simulink model "IEEE9_16b_Rockefeller_uderen"  (R2020a)
settings: Solver=ode8  StartTime=0.0  StopTime=5  MaxStep=1e-4  RelTol=1e-3
undefined symbols (not defined in the file or in its folder): k
libraries: powerlib x33, powerlib_meascontrol x27, simulink_extras x24, dspsigops x6, sps_avr x3
(part 1 of 2)
settings Model: Creator=Pankaj  LastModifiedBy=ahmed
settings DataIOCC: ReturnWorkspaceOutputs=off
settings DebuggingCC: UnconnectedInputMsg=none  UnconnectedOutputMsg=none  UnconnectedLineMsg=none  ArithmeticOperatorsInVariantConditions=warning
settings SFSimCC: SimUseLocalCustomCode=off  CustomCodeUndefinedFunction=UseInterfaceOnly
settings RTWCC: RTWUseLocalCustomCode=off
settings CodeAppCC: StateflowObjectComments=on
settings SimscapeCC: SimscapeNormalizeSystem=off

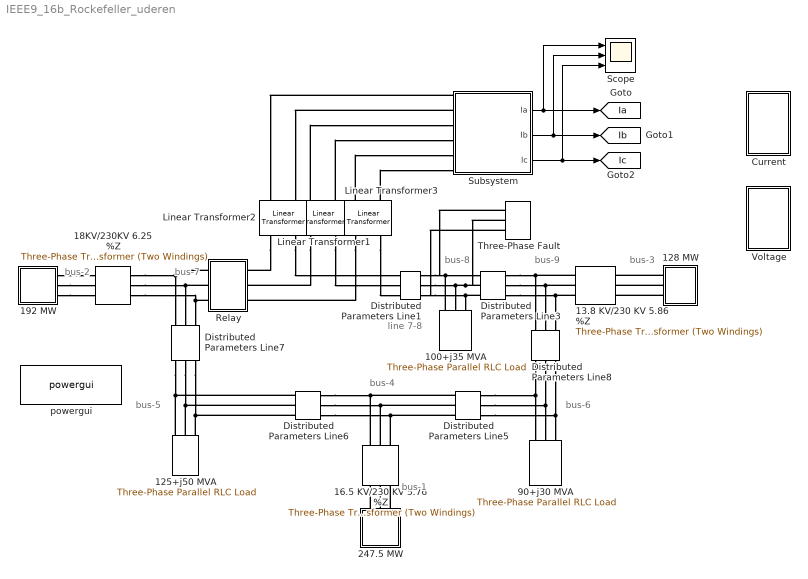
== system IEEE9_16b_Rockefeller_uderen ==
  note: bus-2
  note: bus-7
  note: bus-8
  note: bus-9
  note: bus-1
  note: bus-3
  note: bus-4
  note: bus-6
  note: bus-5
  note: line 7-8
  100+j35 MVA : powerlib/Elements/Three-Phase Parallel RLC Load  LConnTagsString=A|B|C  Configuration=Y (grounded)  NominalVoltage=(230000)*0.993698  Vabc=[1e3 1e3 1e3]  Vabcp=[1e3 1e3 1e3]  NominalFrequency=60  UnbalancedPower=off  ActivePower=100e6  InductivePower=35e6  CapacitivePower=0  Pabc=[10e3 9e3 11e3]  QLabc=[100 90 110]  QCabc=[100 90 110]  Pabcp=[10e3 9e3 11e3]  QLabcp=[100 90 110]  QCabcp=[100 90 110]  Measurements=None  LoadType=constant PQ
  125+j50 MVA : powerlib/Elements/Three-Phase Parallel RLC Load  LConnTagsString=A|B|C  Configuration=Y (grounded)  NominalVoltage=(223027)*1  Vabc=[1e3 1e3 1e3]  Vabcp=[1e3 1e3 1e3]  NominalFrequency=60  UnbalancedPower=off  ActivePower=125e6  InductivePower=50e6  CapacitivePower=0  Pabc=[10e3 9e3 11e3]  QLabc=[100 90 110]  QCabc=[100 90 110]  Pabcp=[10e3 9e3 11e3]  QLabcp=[100 90 110]  QCabcp=[100 90 110]  Measurements=None  LoadType=constant PQ
  128 MW : Subsystem
  13.8 KV/230 KV 5.86 %Z : powerlib/Elements/Three-Phase Transformer (Two Windings)  Winding1Connection=Yg  Winding2Connection=Yg  CoreType=Three single-phase transformers  SetSaturation=off  Hysteresis=off  DataFile='hysteresis'  SetInitialFlux=off  Measurements=None  UNITS=pu  NominalPower=[ 100e6 , 60 ]  Winding1=[13.8e3 , 1e-6 , 0 ]  Winding2=[ 230e3 , 1e-6, 0.0586 ]  Rm=500  Lm=500  L0=0.5  Saturation=[ 0,0 ; 0.0024,1.2 ; 1.0,1.52 ]  InitialFluxes=[ 0.8 , -0.8 , 0.7 ]  BreakLoop=off  DiscreteSolver=Trapezoidal iterative  DataType=off  TransfoNumber=1
  "16.5 KV/230 KV 5.76 %Z     " : powerlib/Elements/Three-Phase Transformer (Two Windings)  Winding1Connection=Yg  Winding2Connection=Yg  CoreType=Three single-phase transformers  SetSaturation=off  Hysteresis=off  DataFile='hysteresis'  SetInitialFlux=off  Measurements=None  UNITS=pu  NominalPower=[ 100e6 , 60 ]  Winding1=[16.5e3 , 1e-6, 0 ]  Winding2=[ 230e3 ,1e-6, 0.0576 ]  Rm=500  Lm=500  L0=0.5  Saturation=[ 0,0 ; 0.0024,1.2 ; 1.0,1.52 ]  InitialFluxes=[ 0.8 , -0.8 , 0.7 ]  BreakLoop=off  DiscreteSolver=Trapezoidal iterative  DataType=off  TransfoNumber=1
  18KV/230KV 6.25 %Z : powerlib/Elements/Three-Phase Transformer (Two Windings)  Winding1Connection=Yg  Winding2Connection=Yg  CoreType=Three single-phase transformers  SetSaturation=off  Hysteresis=off  DataFile='hysteresis'  SetInitialFlux=off  Measurements=None  UNITS=pu  NominalPower=[ 100e6 , 60 ]  Winding1=[ 18e3 , 1e-6 , 0]  Winding2=[ 230e3 , 1e-6, 0.0625 ]  Rm=500  Lm=500  L0=0.5  Saturation=[ 0,0 ; 0.0024,1.2 ; 1.0,1.52 ]  InitialFluxes=[ 0.8 , -0.8 , 0.7 ]  BreakLoop=off  DiscreteSolver=Trapezoidal iterative  DataType=off  TransfoNumber=1
  192 MW : Subsystem
  247.5 MW : Subsystem
  90+j30 MVA : powerlib/Elements/Three-Phase Parallel RLC Load  LConnTagsString=A|B|C  Configuration=Y (grounded)  NominalVoltage=(226177)*0.999999  Vabc=[1e3 1e3 1e3]  Vabcp=[1e3 1e3 1e3]  NominalFrequency=60  UnbalancedPower=off  ActivePower=90e6  InductivePower=30e6  CapacitivePower=0  Pabc=[10e3 9e3 11e3]  QLabc=[100 90 110]  QCabc=[100 90 110]  Pabcp=[10e3 9e3 11e3]  QLabcp=[100 90 110]  QCabcp=[100 90 110]  Measurements=None  LoadType=constant PQ
  "Current " : Subsystem
  Distributed Parameters Line1 : powerlib/Elements/Distributed Parameters Line  Phases=3  Frequency=60  Resistance=[0.044965 0.11241]  Inductance="[1.01e-3  2.02e-3]"  Capacitance=[12.74e-9 7.751e-9]  Length=100  x1=[-0.000416666666666667 4.03999386636865e-10 0 0;-0.000388888888888889 4.03567307365848e-10 0 0;-0.000361111111111111 4.03090972391788e-10 75770.798481712 -217642.762175141;-0.000333333333333333 4.02570433950183e-10 78045.7469011949 -216837.371769227;-0.000305555555555556 4.02005749123939e-10 80312.1367250346 -216008.202701964;-0.000277777777777778 4.0139697983711e-10 82569.7194180468 -215155.345901084;-0.00025 4.0074419284811e-10 84818.2474108487 -214278.894891945;-0.000222222222222222 4.00047459742387e-10 87057.4741270072 -213378.945787278;-0.000194444444444444 3.99306856924578e-10 89287.1540100791 -212455.597276643;-0.000166666666666667 3.98522465610128e-10 91507.042550539 -211508.950615609;-0.000138888888888889 3.97694371816383e-10 93716.8963125926 -210539.109614652;-0.000111111111111111 3.96822666353162e-10 95916.4729608721 -209546.180627764;-8.33333333333333e-05 3.95907444812789e-10 98105.5312870111 -208530.272540801;-5.55555555555556e-05 3.94948807559621e-10 100283.831236096 -207491.49675953;-2.77777777777778e-05 3.93946859719036e-10 102451.133932989 -206429.967197424]  x2=[-0.000416666666666667 2.24406788779024e-10 0 0;-0.000388888888888889 2.22220992142664e-10 0 0;-0.000361111111111111 2.20010826470313e-10 65495.6415441537 -218920.534617487;-0.000333333333333333 2.17776534131542e-10 67784.5337476624 -218222.674162098;-0.000305555555555556 2.15518360141686e-10 70065.9926131833 -217500.88313134;-0.000277777777777778 2.13236552134969e-10 72339.7679530423 -216755.240677735;-0.00025 2.10931360337352e-10 74605.6104221501 -215985.82856938;-0.000222222222222222 2.08603037539095e-10 76863.2715453463 -215192.731180984;-0.000194444444444444 2.06251839067028e-10 79112.5037446472 -214376.035484611;-0.000166666666666667 2.03878022756561e-10 81353.0603663957 -213535.83104015;-0.000138888888888889 2.01481848923403e-10 83584.6957083093 -212672.209985485;-0.000111111111111111 1.99063580335015e-10 85807.1650464246 -211785.267026397;-8.33333333333333e-05 1.96623482181802e-10 88020.2246619337 -210875.099426176;-5.55555555555556e-05 1.94161822048021e-10 90223.6318679107 -209941.806994957;-2.77777777777778e-05 1.91678869882449e-10 92417.1450359256 -208985.492078772]  x3=[-0.000416666666666667 2.4657287812106e-12 0 0;-0.000388888888888889 2.44181675130627e-12 0 0;-0.000361111111111111 2.41763694867838e-12 149.88034762837 -520.868275171293;-0.000333333333333333 2.39319202491478e-12 155.326551453273 -519.270203705918;-0.000305555555555556 2.36848466067682e-12 160.755721971439 -517.615188411064;-0.000277777777777778 2.34351756540542e-12 166.167263813138 -515.903410777807;-0.00025 2.31829347702393e-12 171.560583541825 -514.135058521855;-0.000222222222222222 2.2928151616379e-12 176.935089719215 -512.310325562961;-0.000194444444444444 2.26708541323171e-12 182.29019297014 -510.429412003656;-0.000166666666666667 2.24110705336223e-12 187.625306047182 -508.492524107308;-0.000138888888888889 2.21488293084937e-12 192.93984389507 -506.499874275502;-0.000111111111111111 2.18841592146368e-12 198.233223714842 -504.451681024747;-8.33333333333333e-05 2.161708927611e-12 203.504865027747 -502.348168962514;-5.55555555555556e-05 2.13476487801416e-12 208.754189738911 -500.189568762605;-2.77777777777778e-05 2.10758672739183e-12 213.980622200724 -497.976117139856]  x4=[-0.000416666666666667 -9.98914374453805e-13 0 0;-0.000388888888888889 -9.81740072469835e-13 0 0;-0.000361111111111111 -9.64458111623713e-13 241.700354629401 -1044.85957766127;-0.000333333333333333 -9.47070387077197e-13 252.628607776882 -1042.27124557573;-0.000305555555555556 -9.29578805590225e-13 263.529157350655 -1039.56861670278;-0.000277777777777778 -9.11985285311819e-13 274.40080798262 -1036.75198741614;-0.00025 -8.94291755569738e-13 285.242367473774 -1033.82166659095;-0.000222222222222222 -8.76500156658907e-13 296.052646924945 -1030.7779755699;-0.000194444444444444 -8.58612439628639e-13 306.830460867171 -1027.62124812802;-0.000166666666666667 -8.40630566068683e-13 317.574627391698 -1024.35183043604;-0.000138888888888889 -8.22556507894113e-13 328.28396827959 -1020.97008102246;-0.000111111111111111 -8.04392247129082e-13 338.957309130937 -1017.47637073421;-8.33333333333333e-05 -7.86139775689477e-13 349.593479493636 -1013.87108269599;-5.55555555555556e-05 -7.67801095164478e-13 360.191312991747 -1010.15461226827;-2.77777777777778e-05 -7.49378216597062e-13 370.749647453402 -1006.3273670039]  x5=0.000395689524753941  V1=[5.416e-10 2.305e+05 2.305e+05;377 377 377;2.885 0.3359 -1.235]  V2=[2.789e-10 2.285e+05 2.285e+05;377 377 377;2.728 0.2916 -1.279]  I1=[3.179e-12 542 542;377 377 377;-1.76 0.2811 -1.29]  I2=[4.124e-12 1072 1072;377 377 377;1.614 0.2282 -1.343]  nHarmo=1  Measurements=None
  Distributed Parameters Line3 : powerlib/Elements/Distributed Parameters Line  Phases=3  Frequency=60  Resistance=[ 0.062951 0.15737]  Inductance="[ 1.414e-3  3.53e-3]"  Capacitance=[12.74e-9 7.751e-9]  Length=100  x1=[-0.000527777777777778 2.32901531654904e-10 0 0;-0.0005 2.30815581018941e-10 0 0;-0.000472222222222222 2.28704318853463e-10 0 0;-0.000444444444444444 2.2656797668216e-10 58586.8788444457 -220869.780420169;-0.000416666666666667 2.24406788779024e-10 60896.5619220916 -220244.16032176;-0.000388888888888889 2.22220992142664e-10 63199.5670054809 -219594.387969246;-0.000361111111111111 2.20010826470313e-10 65495.6415441537 -218920.534617487;-0.000333333333333333 2.17776534131542e-10 67784.5337476624 -218222.674162098;-0.000305555555555556 2.15518360141686e-10 70065.9926131833 -217500.88313134;-0.000277777777777778 2.13236552134969e-10 72339.7679530423 -216755.240677735;-0.00025 2.10931360337352e-10 74605.6104221501 -215985.82856938;-0.000222222222222222 2.08603037539095e-10 76863.2715453463 -215192.731180984;-0.000194444444444444 2.06251839067028e-10 79112.5037446472 -214376.035484611;-0.000166666666666667 2.03878022756561e-10 81353.0603663957 -213535.83104015;-0.000138888888888889 2.01481848923403e-10 83584.6957083093 -212672.209985485;-0.000111111111111111 1.99063580335015e-10 85807.1650464246 -211785.267026397;-8.33333333333333e-05 1.96623482181802e-10 88020.2246619337 -210875.099426176;-5.55555555555556e-05 1.94161822048021e-10 90223.6318679107 -209941.806994957;-2.77777777777778e-05 1.91678869882449e-10 92417.1450359256 -208985.492078772]  x2=[-0.000527777777777778 3.2700270716933e-10 0 0;-0.0005 3.25421192626044e-10 0 0;-0.000472222222222222 3.23803991981823e-10 0 0;-0.000444444444444444 3.22151282580942e-10 67656.3360068027 -221170.891319713;-0.000416666666666667 3.20463245661611e-10 69968.6747078772 -220450.281883491;-0.000388888888888889 3.187400663361e-10 72273.3405552948 -219705.497589611;-0.000361111111111111 3.16981933570442e-10 74570.0808164739 -218936.620112065;-0.000333333333333333 3.15189040163706e-10 76858.6436279632 -218143.733766932;-0.000305555555555556 3.13361582726859e-10 79138.7780230604 -217326.925503135;-0.000277777777777778 3.11499761661201e-10 81410.2339593343 -216486.284892905;-0.00025 3.09603781136394e-10 83672.7623460448 -215621.904121957;-0.000222222222222222 3.07673849068068e-10 85926.1150714576 -214733.877979385;-0.000194444444444444 3.05710177095022e-10 88170.0450300536 -213822.303847261;-0.000166666666666667 3.03712980556018e-10 90404.3061496259 -212887.281689962;-0.000138888888888889 3.01682478466161e-10 92628.6534182649 -211928.914043204;-0.000111111111111111 2.99618893492888e-10 94842.8429112266 -210947.306002799;-8.33333333333333e-05 2.97522451931545e-10 97046.6318176814 -209942.565213131;-5.55555555555556e-05 2.95393383680575e-10 99239.7784673413 -208914.80185535;-2.77777777777778e-05 2.93231922216303e-10 101422.042356962 -207864.12863529]  x3=[-0.000527777777777778 5.83625832453338e-13 0 0;-0.0005 5.86026533236036e-13 0 0;-0.000472222222222222 5.88362969605446e-13 0 0;-0.000444444444444444 5.90634885344991e-13 134.791474574619 -835.193347915332;-0.000416666666666667 5.92842031313507e-13 143.530042644098 -833.736052248476;-0.000388888888888889 5.94984165472567e-13 152.252871026964 -832.18732802814;-0.000361111111111111 5.97061052913021e-13 160.959003166788 -830.547345089386;-0.000333333333333333 5.99072465880757e-13 169.647484338072 -828.816283274826;-0.000305555555555556 6.01018183801675e-13 178.317361750944 -826.994332414893;-0.000277777777777778 6.02897993305881e-13 186.967684655647 -825.081692307033;-0.00025 6.04711688251078e-13 195.597504446793 -823.078572693785;-0.000222222222222222 6.06459069745176e-13 204.205874767392 -820.985193239789;-0.000194444444444444 6.08139946168105e-13 212.791851612633 -818.801783507692;-0.000166666666666667 6.09754133192822e-13 221.354493433398 -816.528582932976;-0.000138888888888889 6.11301453805529e-13 229.892861239519 -814.165840797701;-0.000111111111111111 6.12781738325086e-13 238.406018702749 -811.713816203167;-8.33333333333333e-05 6.14194824421613e-13 246.893032259436 -809.172778041503;-5.55555555555556e-05 6.15540557134295e-13 255.352971212904 -806.543004966179;-2.77777777777778e-05 6.16818788888377e-13 263.784907835512 -803.824785361446]  x4=[-0.000527777777777778 7.12462384982262e-13 0 0;-0.0005 7.0072342704295e-13 0 0;-0.000472222222222222 6.88907626883427e-13 0 0;-0.000444444444444444 6.77016280239333e-13 133.427230259186 -503.056878765156;-0.000416666666666667 6.6505069113083e-13 138.687791245764 -501.632070106391;-0.000388888888888889 6.53012171719605e-13 143.933143553162 -500.15225183826;-0.000361111111111111 6.40902042164973e-13 149.16271196939 -498.61758623951;-0.000333333333333333 6.28721630479108e-13 154.375923013341 -497.028241603521;-0.000305555555555556 6.16472272381411e-13 159.572204997674 -495.38439221984;-0.000277777777777778 6.04155311152038e-13 164.750988091513 -493.686218355078;-0.00025 5.91772097484584e-13 169.911704382934 -491.933906233135;-0.000222222222222222 5.79323989337977e-13 175.053787941238 -490.127648014782;-0.000194444444444444 5.6681235178755e-13 180.176674879018 -488.267641776588;-0.000166666666666667 5.54238556875355e-13 185.279803413991 -486.354091489197;-0.000138888888888889 5.41603983459698e-13 190.362613930605 -484.387206994961;-0.000111111111111111 5.28910017063932e-13 195.424549041411 -482.367203984931;-8.33333333333333e-05 5.16158049724521e-13 200.465053648179 -480.2943039752;-5.55555555555556e-05 5.03349479838386e-13 205.483575002779 -478.168734282613;-2.77777777777778e-05 4.90485712009553e-13 210.479562767791 -475.99072799984]  x5=0.000523077718890797  V1=[2.541e-10 2.285e+05 2.285e+05;377 377 377;2.713 0.2668 -1.304]  V2=[4.31e-10 2.313e+05 2.313e+05;377 377 377;2.564 0.3044 -1.266]  I1=[1.418e-12 846 846;377 377 377;1.513 0.1676 -1.403]  I2=[2.062e-12 520.4 520.5;377 377 377;-2.991 0.2668 -1.304]  nHarmo=1  Measurements=None
  Distributed Parameters Line5 : powerlib/Elements/Distributed Parameters Line  Phases=3  Frequency=60  Resistance=[ 0.08993 0.224825]  Inductance="[ 1.29e-3  3.22e-3]"  Capacitance=[12.74e-9 7.751e-9]  Length=100  x1=[-0.0005 1.0080475529374e-10 59236.9573250748 -221110.335723773;-0.000472222222222222 9.85184782910845e-11 61549.1238482215 -220477.894229562;-0.000444444444444444 9.62213976270818e-11 63854.5408163426 -219821.274849687;-0.000416666666666667 9.39137652025128e-11 66152.955414488 -219140.549589866;-0.000388888888888889 9.15958340752774e-11 68444.1155955961 -218435.793099292;-0.000361111111111111 8.92678584326443e-11 70727.7701081341 -217707.082662457;-0.000333333333333333 8.69300935633769e-11 73003.6685236502 -216954.498190672;-0.000305555555555556 8.4582795829737e-11 75271.5612642361 -216178.122213305;-0.000277777777777778 8.2226222639373e-11 77531.199629896 -215378.039868732;-0.00025 7.98606324170912e-11 79782.3358258193 -214554.338894998;-0.000222222222222222 7.74862845765174e-11 82024.722989554 -213707.109620196;-0.000194444444444444 7.51034394916487e-11 84258.1152180784 -212836.444952564;-0.000166666666666667 7.2712358468301e-11 86482.2675947664 -211942.440370294;-0.000138888888888889 7.03133037154533e-11 88696.9362162461 -211025.193911063;-0.000111111111111111 6.79065383164944e-11 90901.878219146 -210084.806161282;-8.33333333333333e-05 6.54923262003719e-11 93096.8518067282 -209121.380245065;-5.55555555555556e-05 6.30709321126501e-11 95281.6162754036 -208135.02181292;-2.77777777777778e-05 6.06426215864773e-11 97455.9320411281 -207125.839030165]  x2=[-0.0005 3.88349738495921e-11 47819.8765851152 -221024.854138414;-0.000472222222222222 3.75142302196108e-11 50131.7738988869 -220511.975319648;-0.000444444444444444 3.6189372731539e-11 52438.1736987168 -219974.914877845;-0.000416666666666667 3.486054667093e-11 54738.8230618762 -219413.731707732;-0.000388888888888889 3.35278977585359e-11 57033.4696962363 -218828.48734937;-0.000361111111111111 3.21915721343275e-11 59321.8619679355 -218219.245981397;-0.000333333333333333 3.08517163414685e-11 61603.7489289732 -217586.074413995;-0.000305555555555556 2.95084773102454e-11 63878.8803447298 -216929.042081562;-0.000277777777777778 2.8162002341955e-11 66147.0067214069 -216248.221035096;-0.00025 2.68124390927508e-11 68407.8793333881 -215543.685934297;-0.000222222222222222 2.54599355574514e-11 70661.2502505137 -214815.514039379;-0.000194444444444444 2.41046400533108e-11 72906.8723652693 -214063.785202596;-0.000166666666666667 2.27467012037536e-11 75144.4994198843 -213288.581859486;-0.000138888888888889 2.13862679220775e-11 77373.8860333364 -212489.989019831;-0.000111111111111111 2.00234893951224e-11 79594.7877282605 -211668.094258336;-8.33333333333333e-05 1.86585150669109e-11 81806.9609577585 -210822.987705023;-5.55555555555556e-05 1.72914946222599e-11 84010.1631321068 -209954.762035348;-2.77777777777778e-05 1.59225779703662e-11 86204.1526453591 -209063.512460042]  x3=[-0.0005 -7.50982334861951e-13 90.1297776583444 -469.287337824947;-0.000472222222222222 -7.61225065980247e-13 95.0391104187908 -468.317788550188;-0.000444444444444444 -7.71384320191832e-13 99.9380210697864 -467.296882952453;-0.000416666666666667 -7.81458983419997e-13 104.825972390573 -466.224732985545;-0.000388888888888889 -7.91447950864387e-13 109.702428362205 -465.101456222789;-0.000361111111111111 -8.01350127122157e-13 114.566854226333 -463.927175844142;-0.000333333333333333 -8.11164426308094e-13 119.418716543844 -462.70202062268;-0.000305555555555556 -8.20889772173693e-13 124.25748325336 -461.426124910478;-0.000277777777777778 -8.30525098225186e-13 129.082623729582 -460.09962862388;-0.00025 -8.40069347840492e-13 133.893608841484 -458.722677228152;-0.000222222222222222 -8.49521474385086e-13 138.689911010332 -457.295421721531;-0.000194444444444444 -8.58880441326777e-13 143.471004267544 -455.818018618667;-0.000166666666666667 -8.68145222349374e-13 148.236364312368 -454.29062993346;-0.000138888888888889 -8.77314801465232e-13 152.985468569372 -452.71342316129;-0.000111111111111111 -8.86388173126671e-13 157.717796245759 -451.086571260654;-8.33333333333333e-05 -8.95364342336239e-13 162.432828388469 -449.410252634196;-5.55555555555556e-05 -9.04242324755831e-13 167.130047941094 -447.684651109143;-2.77777777777778e-05 -9.13021146814629e-13 171.808939800579 -445.909955917148]  x4=[-0.0005 1.03748190399177e-12 134.355884883261 -916.40247338539;-0.000472222222222222 1.03354240972687e-12 143.944855500255 -914.945276234842;-0.000444444444444444 1.02948957588978e-12 153.518040941732 -913.387745024259;-0.000416666666666667 1.02532384691939e-12 163.074391400029 -911.73005055449;-0.000388888888888889 1.02104567963485e-12 172.612858913627 -909.972374610413;-0.000361111111111111 1.01665554318539e-12 182.132397482076 -908.114909941004;-0.000333333333333333 1.01215391899896e-12 191.631963180695 -906.157860238195;-0.000305555555555556 1.00754130072936e-12 201.110514275055 -904.10144011454;-0.000277777777777778 1.00281819420219e-12 210.567011335215 -901.945875079679;-0.00025 9.97985117359288e-13 220.000417349708 -899.69140151561;-0.000222222222222222 9.93042600201997e-13 229.40969783926 -897.338266650764;-0.000194444444444444 9.8799118473302e-13 238.793820970231 -894.886728532896;-0.000166666666666667 9.8283142489699e-13 248.15175766777 -892.337056000788;-0.000138888888888889 9.77563886519715e-13 257.482481728666 -889.689528654765;-0.000111111111111111 9.7218914724614e-13 266.784969933876 -886.944436826035;-8.33333333333333e-05 9.66707796476994e-13 276.058202160739 -884.102081544852;-5.55555555555556e-05 9.61120435304157e-13 285.301161494842 -881.162774507502;-2.77777777777778e-05 9.55427676444746e-13 294.512834341536 -878.126838042126]  x5=0.000499582025297148  V1=[3.29e-10 2.289e+05 2.289e+05;377 377 377;2.341 0.2974 -1.273]  V2=[3.35e-10 2.261e+05 2.261e+05;377 377 377;2.353 0.2487 -1.322]  I1=[9.5e-13 477.9 477.9;377 377 377;2.529 0.2254 -1.345]  I2=[6.245e-14 926.2 926.2;377 377 377;-2.223 0.1812 -1.39]  nHarmo=1  Measurements=None
  Distributed Parameters Line6 : powerlib/Elements/Distributed Parameters Line  Phases=3  Frequency=60  Resistance=[ 0.0529 0.13225]  Inductance="[ 1.192e-3  2.38e-3]"  Capacitance=[12.74e-9 7.751e-9]  Length=100  x1=[-0.000444444444444444 2.06940842119763e-10 0 0;-0.000416666666666667 2.06909650746566e-10 51040.896855504 -217071.807600682;-0.000388888888888889 2.06855769398504e-10 53311.2223029157 -216525.415158399;-0.000361111111111111 2.06779203984275e-10 55575.7015740392 -215955.278264325;-0.000333333333333333 2.06679962900139e-10 57834.0863432037 -215361.459440394;-0.000305555555555556 2.06558057029e-10 60086.1289530699 -214744.023805532;-0.000277777777777778 2.0641349973921e-10 62331.5824417872 -214103.039068515;-0.00025 2.06246306883104e-10 64570.2005700766 -213438.575520542;-0.000222222222222222 2.06056496795265e-10 66801.7378482336 -212750.706027529;-0.000194444444444444 2.05844090290506e-10 69025.9495630483 -212039.506022118;-0.000166666666666667 2.05609110661594e-10 71242.5918046417 -211305.053495403;-0.000138888888888889 2.05351583676695e-10 73451.4214932126 -210547.428988381;-0.000111111111111111 2.05071537576543e-10 75652.1964056946 -209766.715583117;-8.33333333333333e-05 2.0476900307135e-10 77844.6752023179 -208962.998893633;-5.55555555555556e-05 2.04444013337433e-10 80028.6174530755 -208136.367056521;-2.77777777777778e-05 2.0409660401358e-10 82203.7836640888 -207286.910721277]  x2=[-0.000444444444444444 9.62213976270818e-11 0 0;-0.000416666666666667 9.39137652025128e-11 66152.955414488 -219140.549589866;-0.000388888888888889 9.15958340752774e-11 68444.1155955961 -218435.793099292;-0.000361111111111111 8.92678584326443e-11 70727.7701081341 -217707.082662456;-0.000333333333333333 8.69300935633769e-11 73003.6685236502 -216954.498190672;-0.000305555555555556 8.4582795829737e-11 75271.5612642361 -216178.122213305;-0.000277777777777778 8.2226222639373e-11 77531.199629896 -215378.039868732;-0.00025 7.98606324170912e-11 79782.3358258193 -214554.338894998;-0.000222222222222222 7.74862845765174e-11 82024.722989554 -213707.109620196;-0.000194444444444444 7.51034394916487e-11 84258.1152180784 -212836.444952564;-0.000166666666666667 7.2712358468301e-11 86482.2675947664 -211942.440370294;-0.000138888888888889 7.03133037154533e-11 88696.9362162461 -211025.193911063;-0.000111111111111111 6.79065383164944e-11 90901.878219146 -210084.806161282;-8.33333333333333e-05 6.54923262003719e-11 93096.8518067282 -209121.380245065;-5.55555555555556e-05 6.30709321126501e-11 95281.6162754036 -208135.02181292;-2.77777777777778e-05 6.06426215864773e-11 97455.9320411281 -207125.839030165]  x3=[-0.000444444444444444 2.52606252839557e-12 0 0;-0.000416666666666667 2.50355358832189e-12 106.434328763548 -1048.02071772117;-0.000388888888888889 2.48077010538477e-12 117.403114042452 -1046.84869549164;-0.000361111111111111 2.45771457804986e-12 128.359024746888 -1045.56187450574;-0.000333333333333333 2.43438953461553e-12 139.300859437786 -1044.16039587789;-0.000305555555555556 2.41079753293566e-12 150.227418219668 -1042.64441329601;-0.000277777777777778 2.38694116013909e-12 161.137502872234 -1041.01409300468;-0.00025 2.36282303234592e-12 172.029916981755 -1039.26961378688;-0.000222222222222222 2.33844579438066e-12 182.903466072278 -1037.41116694444;-0.000194444444444444 2.31381211948216e-12 193.756957736612 -1035.43895627697;-0.000166666666666667 2.28892470901046e-12 204.589201767087 -1033.35319805962;-0.000138888888888889 2.26378629215058e-12 215.399010286077 -1031.15412101926;-0.000111111111111111 2.23839962561322e-12 226.185197876264 -1028.84196630948;-8.33333333333333e-05 2.21276749333244e-12 236.946581710628 -1026.41698748411;-5.55555555555556e-05 2.18689270616039e-12 247.681981682162 -1023.87945046938;-2.77777777777778e-05 2.16077810155906e-12 258.390220533283 -1021.22963353484]  x4=[-0.000444444444444444 -2.1772534938916e-12 0 0;-0.000416666666666667 -2.16577850452982e-12 167.718963926061 -387.614906849841;-0.000388888888888889 -2.1540660131489e-12 171.768779514311 -385.837332819023;-0.000361111111111111 -2.14211730415553e-12 175.799758720228 -384.01744737667;-0.000333333333333333 -2.12993368786029e-12 179.811459501519 -382.155450093728;-0.000305555555555556 -2.11751650033401e-12 183.803441929985 -380.251545159184;-0.000277777777777778 -2.10486710326122e-12 187.775268239766 -378.305941357667;-0.00025 -2.09198688379086e-12 191.726502875349 -376.31885204656;-0.000222222222222222 -2.07887725438414e-12 195.656712539332 -374.290495132598;-0.000194444444444444 -2.06553965265967e-12 199.565466239933 -372.221093047974;-0.000166666666666667 -2.05197554123576e-12 203.452335338263 -370.110872725947;-0.000138888888888889 -2.0381864075701e-12 207.316893595324 -367.960065575955;-0.000111111111111111 -2.02417376379657e-12 211.158717218753 -365.768907458239;-8.33333333333333e-05 -2.00993914655948e-12 214.977384909296 -363.53763865798;-5.55555555555556e-05 -1.99548411684501e-12 218.772477907009 -361.266503858946;-2.77777777777778e-05 -1.98081025981006e-12 222.543580037178 -358.955752116659]  x5=0.000429504132692574  V1=[5.692e-10 2.23e+05 2.23e+05;377 377 377;2.022 0.2411 -1.33]  V2=[3.29e-10 2.289e+05 2.289e+05;377 377 377;2.367 0.3033 -1.267]  I1=[3.839e-12 1053 1053;377 377 377;3.112 0.1114 -1.459]  I2=[2.337e-12 422.3 422.3;377 377 377;0.2722 0.4185 -1.152]  nHarmo=1  Measurements=None
  Distributed Parameters Line7 : powerlib/Elements/Distributed Parameters Line  Phases=3  Frequency=60  Resistance=[ 0.16928 0.4232]  Inductance="[ 2.259e-3  5.64e-3]"  Capacitance=[12.74e-9 7.751e-9]  Length=100  x1=[-0.000666666666666667 2.06373646123582e-10 30386.1592924957 -220911.816974351;-0.000638888888888889 2.06523888667017e-10 32697.828929352 -220581.506414806;-0.000611111111111111 2.06651483538748e-10 35005.9128807952 -220227.006607356;-0.000583333333333333 2.06756416746558e-10 37310.1580394103 -219848.356426898;-0.000555555555555556 2.06838676783339e-10 39610.311718749 -219445.597396692;-0.000527777777777778 2.0689825462835e-10 41906.1216810402 -219018.773683804;-0.0005 2.0693514374821e-10 44197.3361648499 -218567.932094265;-0.000472222222222222 2.06949340097611e-10 46483.7039126905 -218093.122067935;-0.000444444444444445 2.06940842119763e-10 48764.9741985733 -217594.395673085;-0.000416666666666667 2.06909650746566e-10 51040.8968555039 -217071.807600682;-0.000388888888888889 2.06855769398504e-10 53311.2223029157 -216525.415158399;-0.000361111111111111 2.06779203984275e-10 55575.7015740391 -215955.278264325;-0.000333333333333333 2.06679962900139e-10 57834.0863432037 -215361.459440394;-0.000305555555555556 2.06558057029e-10 60086.1289530699 -214744.023805532;-0.000277777777777778 2.0641349973921e-10 62331.5824417872 -214103.039068515;-0.00025 2.06246306883104e-10 64570.2005700766 -213438.575520542;-0.000222222222222222 2.06056496795265e-10 66801.7378482336 -212750.706027529;-0.000194444444444444 2.05844090290506e-10 69025.9495630483 -212039.506022118;-0.000166666666666667 2.05609110661594e-10 71242.5918046417 -211305.053495403;-0.000138888888888889 2.05351583676695e-10 73451.4214932126 -210547.428988381;-0.000111111111111111 2.05071537576543e-10 75652.1964056946 -209766.715583117;-8.33333333333333e-05 2.0476900307135e-10 77844.6752023179 -208962.998893633;-5.55555555555556e-05 2.04444013337433e-10 80028.6174530755 -208136.367056521;-2.77777777777778e-05 2.0409660401358e-10 82203.7836640888 -207286.910721277]  x2=[-0.000666666666666667 4.20651827920602e-10 50253.4640487239 -224909.288392932;-0.000638888888888889 4.22467741272632e-10 52605.9049579797 -224370.712165158;-0.000611111111111111 4.24237326276052e-10 54952.5770369422 -223807.531160367;-0.000583333333333333 4.25960388875926e-10 57293.2229465733 -223219.807137703;-0.000555555555555556 4.27636740119023e-10 59627.5860086724 -222607.604547727;-0.000527777777777778 4.29266196174537e-10 61955.4102340239 -221970.990525353;-0.0005 4.3084857835425e-10 64276.4403504691 -221310.034882482;-0.000472222222222222 4.32383713132125e-10 66590.4218309003 -220624.810100349;-0.000444444444444445 4.33871432163333e-10 68897.1009211719 -219915.391321572;-0.000416666666666667 4.35311572302718e-10 71196.2246679277 -219181.856341917;-0.000388888888888889 4.36703975622685e-10 73487.5409463401 -218424.285601758;-0.000361111111111111 4.38048489430517e-10 75770.7984877585 -217642.762177265;-0.000333333333333333 4.39344966285126e-10 78045.7469072634 -216837.371771288;-0.000305555555555556 4.40593264013214e-10 80312.1367311243 -216008.202703961;-0.000277777777777778 4.41793245724869e-10 82569.7194241571 -215155.345903017;-0.00025 4.42944779828572e-10 84818.2474169788 -214278.894893814;-0.000222222222222222 4.44047740045632e-10 87057.4741331566 -213378.945789083;-0.000194444444444444 4.45102005424034e-10 89287.154016247 -212455.597278383;-0.000166666666666667 4.46107460351697e-10 91507.0425567248 -211508.950617285;-0.000138888888888889 4.47063994569159e-10 93716.8963187957 -210539.109616262;-0.000111111111111111 4.47971503181663e-10 95916.4729670917 -209546.18062931;-8.33333333333333e-05 4.48829886670662e-10 98105.5312932465 -208530.272542281;-5.55555555555556e-05 4.49639050904736e-10 100283.831242346 -207491.496760945;-2.77777777777778e-05 4.50398907149906e-10 102451.133939254 -206429.967198773]  x3=[-0.000666666666666667 -3.57088859299639e-13 16.9125422075388 -746.512553780918;-0.000638888888888889 -3.44840348732127e-13 24.7289171507432 -746.294517289108;-0.000611111111111111 -3.32554022534378e-13 32.5425802895125 -745.994641193502;-0.000583333333333333 -3.20231228040516e-13 40.3526747676315 -745.612958378894;-0.000555555555555556 -3.07873316583821e-13 48.1583441202289 -745.149510701105;-0.000527777777777778 -2.95481643348546e-13 55.9587323676983 -744.604348982397;-0.0005 -2.83057567221302e-13 63.752984109566 -743.977533005894;-0.000472222222222222 -2.70602450642044e-13 71.5402446182952 -743.269131509032;-0.000444444444444445 -2.5811765945466e-13 79.3196599330168 -742.479222176018;-0.000416666666666667 -2.45604562757195e-13 87.0903769531753 -741.607891629312;-0.000388888888888889 -2.33064532751712e-13 94.8515435320816 -740.655235420128;-0.000361111111111111 -2.20498944593814e-13 102.60230857036 -739.621358017954;-0.000333333333333333 -2.07909176241845e-13 110.341822109281 -738.506372799099;-0.000305555555555556 -1.95296608305777e-13 118.069235423968 -737.310402034256;-0.000277777777777778 -1.82662623895815e-13 125.783701116471 -736.033576875096;-0.00025 -1.70008608470723e-13 133.484373208694 -734.676037339888;-0.000222222222222222 -1.57335949685889e-13 141.170407235162 -733.237932298138;-0.000194444444444444 -1.44646037241157e-13 148.84096033563 -731.719419454272;-0.000166666666666667 -1.31940262728428e-13 156.495191347513 -730.120665330335;-0.000138888888888889 -1.1922001947906e-13 164.132260898124 -728.441845247732;-0.000111111111111111 -1.06486702411069e-13 171.751331496725 -726.683143308004;-8.33333333333333e-05 -9.37417078761619e-14 179.351567626366 -724.844752372637;-5.55555555555556e-05 -8.09864335066133e-14 186.932135835509 -722.926874041915;-2.77777777777778e-05 -6.82222780619966e-14 194.492204829423 -720.929718632809]  x4=[-0.000666666666666667 7.35770515887366e-13 63.6030871374714 -299.765578932973;-0.000638888888888889 7.25568530046539e-13 66.7386721330621 -299.083104234926;-0.000611111111111111 7.15286977439979e-13 69.8669384811769 -298.367831704139;-0.000583333333333333 7.04926985555791e-13 72.9875431321584 -297.619839778306;-0.000555555555555556 6.94489690483832e-13 76.1001438765406 -296.839210483171;-0.000527777777777778 6.83976236791123e-13 79.2043993825761 -296.026029423532;-0.0005 6.73387777396339e-13 82.2999692336668 -295.180385773857;-0.000472222222222222 6.62725473443373e-13 85.3865139656946 -294.302372268501;-0.000444444444444445 6.51990494174006e-13 88.4636951042476 -293.39208519154;-0.000416666666666667 6.41184016799689e-13 91.5311752017372 -292.449624366209;-0.000388888888888889 6.30307226372441e-13 94.5886178744033 -291.475093143959;-0.000361111111111111 6.19361315654906e-13 97.6356878392027 -290.468598393119;-0.000333333333333333 6.08347484989541e-13 100.672050950576 -289.430250487183;-0.000305555555555556 5.97266942166994e-13 103.697374237092 -288.360163292697;-0.000277777777777778 5.86120902293652e-13 106.71132593796 -287.258454156784;-0.00025 5.74910587658391e-13 109.713575539411 -286.125243894263;-0.000222222222222222 5.6363722759854e-13 112.703793810945 -284.960656774411;-0.000194444444444444 5.52302058365068e-13 115.681652841431 -283.764820507329;-0.000166666666666667 5.40906322987018e-13 118.646826075069 -282.537866229939;-0.000138888888888889 5.29451271135193e-13 121.5989883472 -281.279928491605;-0.000111111111111111 5.17938158985114e-13 124.537815919963 -279.991145239375;-8.33333333333333e-05 5.06368249079269e-13 127.462986517796 -278.671657802856;-5.55555555555556e-05 4.94742810188662e-13 130.37417936278 -277.321610878715;-2.77777777777778e-05 4.83063117173673e-13 133.271075209814 -275.94115251481]  x5=0.000661178039562719  V1=[5.692e-10 2.23e+05 2.23e+05;377 377 377;1.934 0.1858 -1.385]  V2=[7.107e-10 2.305e+05 2.305e+05;377 377 377;2.15 0.2689 -1.302]  I1=[1.362e-12 746.7 746.7;377 377 377;1.537 0.07174 -1.499]  I2=[6.286e-13 306.4 306.4;377 377 377;-2.668 0.2582 -1.313]  nHarmo=1  Measurements=None
  Distributed Parameters Line8 : powerlib/Elements/Distributed Parameters Line  Phases=3  Frequency=60  Resistance=[ 0.20631 0.5157]  Inductance="[ 2.38e-3  6.09e-3]"  Capacitance=[12.74e-9 7.751e-9]  Length=100  x1=[-0.000694444444444444 4.79528859754174e-11 0 0;-0.000666666666666667 4.66649674579432e-11 0 0;-0.000638888888888889 4.53719316009209e-11 0 0;-0.000611111111111111 4.40739202003033e-11 0 0;-0.000583333333333333 4.27710755976678e-11 0 0;-0.000555555555555556 4.14635406646068e-11 43180.6040931817 -221977.844593019;-0.000527777777777778 4.01514587870604e-11 45502.735282995 -221513.4950912;-0.0005 3.88349738495921e-11 47819.8765851152 -221024.854138414;-0.000472222222222222 3.75142302196108e-11 50131.7738988869 -220511.975319648;-0.000444444444444444 3.6189372731539e-11 52438.1736987168 -219974.914877845;-0.000416666666666667 3.486054667093e-11 54738.8230618762 -219413.731707732;-0.000388888888888889 3.35278977585359e-11 57033.4696962363 -218828.48734937;-0.000361111111111111 3.21915721343275e-11 59321.8619679355 -218219.245981398;-0.000333333333333333 3.08517163414685e-11 61603.7489289732 -217586.074413995;-0.000305555555555556 2.95084773102454e-11 63878.8803447298 -216929.042081562;-0.000277777777777778 2.8162002341955e-11 66147.0067214069 -216248.221035096;-0.00025 2.68124390927508e-11 68407.8793333881 -215543.685934297;-0.000222222222222222 2.54599355574514e-11 70661.2502505137 -214815.514039379;-0.000194444444444444 2.41046400533108e-11 72906.8723652693 -214063.785202596;-0.000166666666666667 2.27467012037536e-11 75144.4994198843 -213288.581859486;-0.000138888888888889 2.13862679220775e-11 77373.8860333364 -212489.989019831;-0.000111111111111111 2.00234893951224e-11 79594.7877282605 -211668.094258336;-8.33333333333333e-05 1.86585150669109e-11 81806.9609577585 -210822.987705023;-5.55555555555556e-05 1.72914946222599e-11 84010.1631321068 -209954.762035348;-2.77777777777778e-05 1.59225779703662e-11 86204.1526453591 -209063.512460042]  x2=[-0.000694444444444444 3.35732950476346e-10 0 0;-0.000666666666666667 3.34369056311887e-10 0 0;-0.000638888888888889 3.32968494812407e-10 0 0;-0.000611111111111111 3.31531419565257e-10 0 0;-0.000583333333333333 3.30057988161932e-10 0 0;-0.000555555555555556 3.28548362180789e-10 58335.3361825088 -223810.039974746;-0.000527777777777778 3.2700270716933e-10 60675.8225617411 -223186.893559915;-0.0005 3.25421192626044e-10 63009.6551532751 -222539.272187116;-0.000472222222222222 3.23803991981823e-10 65336.5780260673 -221867.246875333;-0.000444444444444444 3.22151282580942e-10 67656.3360068027 -221170.891319713;-0.000416666666666667 3.20463245661611e-10 69968.6747078772 -220450.281883491;-0.000388888888888889 3.187400663361e-10 72273.3405552948 -219705.497589611;-0.000361111111111111 3.16981933570442e-10 74570.0808164739 -218936.620112065;-0.000333333333333333 3.15189040163706e-10 76858.6436279632 -218143.733766932;-0.000305555555555556 3.13361582726859e-10 79138.7780230604 -217326.925503135;-0.000277777777777778 3.11499761661201e-10 81410.2339593343 -216486.284892905;-0.00025 3.09603781136394e-10 83672.7623460448 -215621.904121957;-0.000222222222222222 3.07673849068068e-10 85926.1150714576 -214733.877979385;-0.000194444444444444 3.05710177095022e-10 88170.0450300536 -213822.303847261;-0.000166666666666667 3.03712980556018e-10 90404.3061496259 -212887.281689962;-0.000138888888888889 3.01682478466161e-10 92628.6534182649 -211928.914043204;-0.000111111111111111 2.99618893492888e-10 94842.8429112266 -210947.306002799;-8.33333333333333e-05 2.97522451931545e-10 97046.6318176814 -209942.565213131;-5.55555555555556e-05 2.95393383680575e-10 99239.7784673413 -208914.80185535;-2.77777777777778e-05 2.93231922216303e-10 101422.042356962 -207864.12863529]  x3=[-0.000694444444444444 6.10636454317108e-13 0 0;-0.000666666666666667 6.20247556486954e-13 0 0;-0.000638888888888889 6.29790641522677e-13 0 0;-0.000611111111111111 6.39264662917461e-13 0 0;-0.000583333333333333 6.48668581738099e-13 0 0;-0.000555555555555556 6.58001366738918e-13 61.0186256200025 -667.844629695412;-0.000527777777777778 6.67261994474873e-13 68.0087989359431 -667.169041730528;-0.0005 6.76449449413775e-13 74.991514320691 -666.420291161907;-0.000472222222222222 6.85562724047656e-13 81.9660060408159 -665.598460098485;-0.000444444444444444 6.94600819003256e-13 88.9315092647056 -664.703638663301;-0.000416666666666667 7.03562743151611e-13 95.8872601464374 -663.735924983608;-0.000388888888888889 7.12447513716749e-13 102.832495909543 -662.695425180117;-0.000361111111111111 7.21254156383454e-13 109.766454930655 -661.582253355356;-0.000333333333333333 7.29981705404117e-13 116.688376823029 -660.39653158116;-0.000305555555555556 7.38629203704635e-13 123.597502519925 -659.138389885284;-0.000277777777777778 7.47195702989373e-13 130.493074357853 -657.807966237142;-0.00025 7.55680263845147e-13 137.374336159654 -656.40540653268;-0.000222222222222222 7.64081955844249e-13 144.240533317427 -654.930864578376;-0.000194444444444444 7.72399857646471e-13 151.090912875279 -653.384502074371;-0.000166666666666667 7.80633057100147e-13 157.924723611894 -651.766488596739;-0.000138888888888889 7.88780651342177e-13 164.741216122915 -650.077001578891;-0.000111111111111111 7.96841746897037e-13 171.539642903124 -648.316226292119;-8.33333333333333e-05 8.04815459774759e-13 178.319258428412 -646.484355825273;-5.55555555555556e-05 8.12700915567872e-13 185.079319237539 -644.581591063595;-2.77777777777778e-05 8.20497249547285e-13 191.819084013656 -642.608140666683]  x4=[-0.000694444444444444 -2.88279407422444e-14 0 0;-0.000666666666666667 -4.11033317732574e-14 0 0;-0.000638888888888889 -5.33742153607489e-14 0 0;-0.000611111111111111 -6.56392458640535e-14 0 0;-0.000583333333333333 -7.78970782843619e-14 0 0;-0.000555555555555556 -9.01463684122162e-14 60.6746926977236 -351.106773937345;-0.000527777777777778 -1.02385772974917e-13 64.3480620013862 -350.452148355656;-0.0005 -1.14613949783828e-13 68.0143748149137 -349.759091746663;-0.000472222222222222 -1.26829557881563e-13 71.6732290857903 -349.027680111834;-0.000444444444444444 -1.39031257689038e-13 75.3242235794138 -348.257993658696;-0.000416666666666667 -1.51217711152367e-13 78.966957923095 -347.450116792042;-0.000388888888888889 -1.633875818896e-13 82.6010326499631 -346.604138104675;-0.000361111111111111 -1.75539535337267e-13 86.2260492427722 -345.720150367691;-0.000333333333333333 -1.87672238896735e-13 89.8416101776025 -344.798250520307;-0.000305555555555556 -1.99784362080333e-13 93.447318967454 -343.838539659231;-0.000277777777777778 -2.11874576657264e-13 97.0427802057251 -342.841123027573;-0.00025 -2.23941556799255e-13 100.627599609574 -341.806110003307;-0.000222222222222222 -2.35983979225951e-13 104.201384063155 -340.733614087274;-0.000194444444444444 -2.48000523350027e-13 107.763741660732 -339.623752890738;-0.000166666666666667 -2.59989871422006e-13 111.314281749648 -338.476648122485;-0.000138888888888889 -2.71950708674764e-13 114.852614973172 -337.29242557548;-0.000111111111111111 -2.8388172346771e-13 118.378353313193 -336.071215113071;-8.33333333333333e-05 -2.95781607430621e-13 121.891110132771 -334.813150654747;-5.55555555555556e-05 -3.07649055607122e-13 125.390500218535 -333.518370161452;-2.77777777777778e-05 -3.19482766597786e-13 128.876139822927 -332.187015620458]  x5=0.000687048688231045  V1=[3.258e-10 2.261e+05 2.261e+05;377 377 377;2.369 0.194 -1.377]  V2=[4.31e-10 2.313e+05 2.313e+05;377 377 377;2.502 0.2568 -1.314]  I1=[9.177e-13 670.6 670.6;377 377 377;2.076 0.09296 -1.478]  I2=[4.71e-13 356.3 356.3;377 377 377;-2.438 0.173 -1.398]  nHarmo=1  Measurements=None
  Linear Transformer1 : powerlib/Elements/Linear Transformer  UNITS=pu  NominalPower=[ 150e8 60 ]  winding1=[1 0.002 1]  winding2=[1 0.002 1]  ThreeWindings=off  winding3=[3.15e+05 0.002 0.079997]  RmLm=[499.99 500]  Measurements=None  DataType=off
  Linear Transformer2 : powerlib/Elements/Linear Transformer  UNITS=pu  NominalPower=[ 150e8 60 ]  winding1=[1 0.002 1]  winding2=[1 0.002 1]  ThreeWindings=off  winding3=[3.15e+05 0.002 0.079997]  RmLm=[499.99 500]  Measurements=None  DataType=off
  Linear Transformer3 : powerlib/Elements/Linear Transformer  UNITS=pu  NominalPower=[ 150e8 60 ]  winding1=[1 0.002 1]  winding2=[1 0.002 1]  ThreeWindings=off  winding3=[3.15e+05 0.002 0.079997]  RmLm=[499.99 500]  Measurements=None  DataType=off
  Relay : Subsystem
  Scope : Scope  NumInputPorts=3
  Subsystem : Subsystem
  Three-Phase Fault : powerlib/Elements/Three-Phase Fault  InitialStates=0  FaultA=on  FaultB=off  FaultC=off  GroundFault=on  SwitchTimes=1  External=off  SwitchStatus=NaN  FaultResistance=1e-9  GroundResistance=0.01  SnubberResistance=1e6  SnubberCapacitance=inf  Measurements=None
  Voltage : Subsystem
  powergui : powerlib/powergui  Priority=1  SimulationMode=Discrete  SampleTime=1/1200/30  frequency=60  Iterations=50  frequencyindice=60  Pbase=100e6  ErrMax=0.0001  UnitsV=kV  UnitsW=MW  buscounter=0  FunctionMessages=off  echomessages=off  EnableUseOfTLC=off  CurrentSourceSwitches=off  DisableSnubberDevices=off  DisableRonSwitches=off  DisableVfSwitches=off  DisplayEquations=off  AutomaticDiscreteSolvers=off  SolverType=Tustin/Backward Euler (TBE)  Interpol=off  ExternalGateDelay=off  methode=off  Ts=100  x0status=blocks  SPID=on  SwTol=0  HookPort=off  NonlinearTolerance=1e-4  nMaxIteration=100  ContinueOnMaxIteration=off  RestoreLinks=warning  ResistiveCurrentMeasurement=off  Frange=[0:2:500]  Ylog=off  Xlog=on  ShowGrid=off  save=off  variable=ZData  structure=0  ZoomFFT=off  StartTime=0.0  cycles=1  DisplayStyle=1  fundamental=60  FreqAxis=off  MaxFrequency=1000  frequencyindicesteady=1  RmsSteady=1  display=off
  tag scope: Ia=global, Ib=global, Ic=global
  wires:
  Subsystem/1(Ia) -> Scope/1, [Ia]
  Subsystem/2(Ib) -> Scope/2, [Ib]
  Subsystem/3(Ic) -> Scope/3, [Ic]
  connections:
  Distributed Parameters Line3/LConn2 -- Distributed Parameters Line1/RConn2 -- 100+j35 MVA/LConn2 -- Three-Phase Fault/LConn2
  Distributed Parameters Line3/LConn3 -- Three-Phase Fault/LConn3 -- Distributed Parameters Line1/RConn3 -- 100+j35 MVA/LConn3
  Distributed Parameters Line5/RConn1 -- Distributed Parameters Line8/LConn1 -- 90+j30 MVA/LConn1
  Distributed Parameters Line5/RConn3 -- Distributed Parameters Line8/LConn3 -- 90+j30 MVA/LConn3
  Distributed Parameters Line6/LConn1 -- Distributed Parameters Line7/LConn1 -- 125+j50 MVA/LConn1
  Distributed Parameters Line6/LConn2 -- Distributed Parameters Line7/LConn2 -- 125+j50 MVA/LConn2
  Distributed Parameters Line6/LConn3 -- Distributed Parameters Line7/LConn3 -- 125+j50 MVA/LConn3
  Distributed Parameters Line3/RConn1 -- 13.8 KV/230 KV 5.86 %Z/RConn1 -- Distributed Parameters Line8/RConn1
  Distributed Parameters Line3/RConn2 -- 13.8 KV/230 KV 5.86 %Z/RConn2 -- Distributed Parameters Line8/RConn2
  Distributed Parameters Line3/RConn3 -- 13.8 KV/230 KV 5.86 %Z/RConn3 -- Distributed Parameters Line8/RConn3
  18KV/230KV 6.25 %Z/RConn1 -- Relay/LConn1 -- Distributed Parameters Line7/RConn1
  18KV/230KV 6.25 %Z/RConn2 -- Relay/LConn2 -- Distributed Parameters Line7/RConn2
  18KV/230KV 6.25 %Z/RConn3 -- Relay/LConn3 -- Distributed Parameters Line7/RConn3
  Distributed Parameters Line5/RConn2 -- Distributed Parameters Line8/LConn2 -- 90+j30 MVA/LConn2
  Distributed Parameters Line6/RConn1 -- "16.5 KV/230 KV 5.76 %Z     "/RConn1 -- Distributed Parameters Line5/LConn1
  Distributed Parameters Line6/RConn2 -- "16.5 KV/230 KV 5.76 %Z     "/RConn2 -- Distributed Parameters Line5/LConn2
  Distributed Parameters Line6/RConn3 -- "16.5 KV/230 KV 5.76 %Z     "/RConn3 -- Distributed Parameters Line5/LConn3
  247.5 MW/RConn1 -- "16.5 KV/230 KV 5.76 %Z     "/LConn1
  247.5 MW/RConn2 -- "16.5 KV/230 KV 5.76 %Z     "/LConn2
  247.5 MW/RConn3 -- "16.5 KV/230 KV 5.76 %Z     "/LConn3
  128 MW/RConn1 -- 13.8 KV/230 KV 5.86 %Z/LConn1
  128 MW/RConn2 -- 13.8 KV/230 KV 5.86 %Z/LConn2
  128 MW/RConn3 -- 13.8 KV/230 KV 5.86 %Z/LConn3
  192 MW/RConn1 -- 18KV/230KV 6.25 %Z/LConn1
  192 MW/RConn2 -- 18KV/230KV 6.25 %Z/LConn2
  192 MW/RConn3 -- 18KV/230KV 6.25 %Z/LConn3
  Subsystem/LConn1 -- Linear Transformer2/RConn1
  Subsystem/LConn2 -- Linear Transformer2/RConn2
  Linear Transformer1/RConn1 -- Subsystem/LConn3
  Linear Transformer1/RConn2 -- Subsystem/LConn4
  Linear Transformer3/RConn1 -- Subsystem/LConn5
  Linear Transformer3/RConn2 -- Subsystem/LConn6
  100+j35 MVA/LConn1 -- Three-Phase Fault/LConn1 -- Distributed Parameters Line1/RConn1 -- Distributed Parameters Line3/LConn1
  Linear Transformer2/LConn1 -- Relay/RConn1
  Linear Transformer2/LConn2 -- Distributed Parameters Line1/LConn1
  Linear Transformer1/LConn1 -- Relay/RConn2
  Linear Transformer1/LConn2 -- Distributed Parameters Line1/LConn2
  Linear Transformer3/LConn1 -- Relay/RConn3
  Linear Transformer3/LConn2 -- Distributed Parameters Line1/LConn3

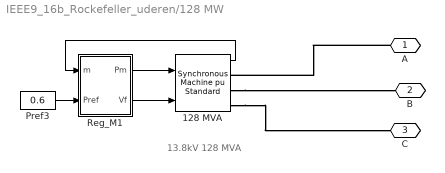
== system IEEE9_16b_Rockefeller_uderen/128 MW ==
  note: 13.8kV 128 MVA
  128 MVA : powerlib/Machines/Synchronous Machine pu Standard  PresetModel=No  MechanicalLoad=Mechanical power Pm  ShowDetailedParameters=on  RotorType=Salient-pole  Units=per unit standard parameters  MeasurementBus=off  NominalParameters="[128e6  13800   60 ]"  Reactances1=[ 31 32 33 34 35 36 37 ]  Reactances2=[ 1.305, 0.296, 0.252, 0.474, 0.243, 0.18 ]  dAxisTimeConstants=Short-circuit  qAxisTimeConstants=Open-circuit  TimeConstants1=[]  TimeConstants2=[]  TimeConstants3=[]  TimeConstants4=[]  TimeConstants5=[ 1.01, 0.053, 0.1 ]  TimeConstants6=[]  TimeConstants7=[]  TimeConstants8=[]  StatorResistance=2.8544e-3  Mechanical="[20 0  32]"  PolePairs=32  InitialConditions=[0 -74.5248 0.603223 0.603223 0.603223 5.08525 -114.915 125.085 1.10339]  SetSaturation=off  Saturation=[0.6404,0.7127,0.8441,0.9214,0.9956,1.082,1.19,1.316,1.457;0.7,0.7698,0.8872,0.9466,0.9969,1.046,1.1,1.151,1.201]  LoadFlowParameters=[1 500000000 0 0 0]  TsPowergui=0  TsBlock=-1  IterativeModel=Trapezoidal non iterative  IterativeDiscreteModel=Trapezoidal non iterative  BusType=PV  Pref=0.6*128e6  Qref=0  Qmin=-Inf  Qmax=Inf  PLF=0  QLF=0
      settings: AttributesFormatString=\n\n
  Pref3 : Constant  Value=0.6
  Reg_M1 : Subsystem
  A : PMIOPort  Side=Right
  B : PMIOPort  Port=2  Side=Right
  C : PMIOPort  Port=3  Side=Right
  wires:
  Reg_M1/1(Pm) -> 128 MVA/1
  Reg_M1/2(Vf) -> 128 MVA/2
  Pref3/1 -> Reg_M1/2(Pref)
  128 MVA/1 -> Reg_M1/1(m)
  connections:
  A/RConn1 -- 128 MVA/RConn1
  128 MVA/RConn2 -- B/RConn1
  128 MVA/RConn3 -- C/RConn1
